simulink model "following_sim"  (R2019b)
settings: Solver=VariableStepAuto  StartTime=0.0  StopTime=10.0  RelTol=1e-3
values from neighbouring files (symbols this model uses):
  A = [0 1 0 0 ... (first row only)    [following.m]    (also in following2.m; observer.m; opt_servo.m; optimal_care.m = [0 1)
  B = [0 ... (first row only)    [following.m]    (also in following2.m; observer.m; opt_servo.m; optimal_care.m)
  C = [0 0 1 0]    [following.m]    (also in following2.m; observer.m; opt_servo.m)
  H = [-K 1]*inv(M0)*[zeros(4,1) ... (first row only)    [following.m]    (also in observer.m; optimal_hamilton.m = [A -B*inv(R)*B')
  K = -acker(A,B,p)    [following.m]    (also in following2.m = Ke(1:4); observer.m; opt_servo.m = -inv(Re)*B'*P11; optimal_care.m = -inv(R)*B'*P)
  x0 = zeros(4,1)    [following.m]    (also in following2.m; observer.m = [-0.5 0 0.5 0]'; opt_servo.m = [ 0 0 0.25 0 ]'; optimal_care.m = [1)
settings Model: Creator=shohei  LastModifiedBy=shohei

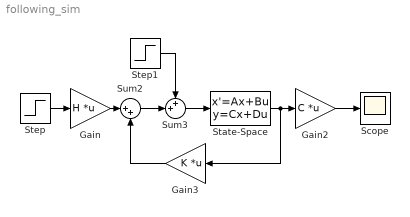
== system following_sim ==
  Gain : Gain  Gain=H  Multiplication=Matrix(K*u)
  Gain2 : Gain  Gain=C  Multiplication=Matrix(K*u)
  Gain3 : Gain  Gain=K  Multiplication=Matrix(K*u)
  Scope : Scope
  State-Space : StateSpace  A=A  B=B  C=eye(4)  D=zeros(4,1)  InitialCondition=x0
  Step : Step  Time=0  SampleTime=0
  Step1 : Step  Time=5  SampleTime=0
  Sum2 : Sum  Inputs=|++
  Sum3 : Sum  Inputs=++|
  wires:
  State-Space/1 -> Gain3/1, Gain2/1
  Gain2/1 -> Scope/1
  Sum3/1 -> State-Space/1
  Step/1 -> Gain/1
  Sum2/1 -> Sum3/2
  Step1/1 -> Sum3/1
  Gain/1 -> Sum2/1
  Gain3/1 -> Sum2/2
